simulink model "LQR_Luenberger_Hardware"  (R2021a)
settings: Solver=FixedStepAuto  StartTime=0.0  StopTime=100  FixedStep=0.002  RelTol=1e-3  EnableMultiTasking=on
undefined symbols (not defined in the file): K_lqr
libraries: simulink_extras x2, cstblocks x1
settings Model: ExtModeTrigDuration=10000  Creator=ACSI-MLC  LastModifiedBy=jameshong
settings SolverCC: AlgebraicLoopSolver=TrustRegion  PositivePriorityOrder=on
settings DataIOCC: ReturnWorkspaceOutputs=off
settings DebuggingCC: SFMachineParentedDataDiag=warning  ArithmeticOperatorsInVariantConditions=warning
settings SFSimCC: CustomCodeUndefinedFunction=UseInterfaceOnly
settings RTWCC: Description=QUARC Win64 Target  SystemTargetFile=quarc_win64.tlc  TemplateMakefile=quarc_default_tmf
settings STFCustomTargetCC: TargetPreCompLibLocation=C:\PROGRA~3\QUARC\lib\2018b\win64\release  TargetLangStandard=C99 (ISO)  ConcurrentExecutionCompliant=on  UseToolchainInfoCompliant=off  SystemTargetFile=quarc_win64.tlc
settings GRTTargetCC: TargetPreCompLibLocation=C:\PROGRA~3\QUARC\lib\2018b\win64\release  ParMdlRefBuildCompliant=off  CompOptLevelCompliant=off  CombineOutputUpdateFcns=off  MatFileLogging=off  CPPClassGenCompliant=off  GRTInterface=on  UseToolchainInfoCompliant=off  ExtMode=on  ExtModeMexFile=quarc_comm

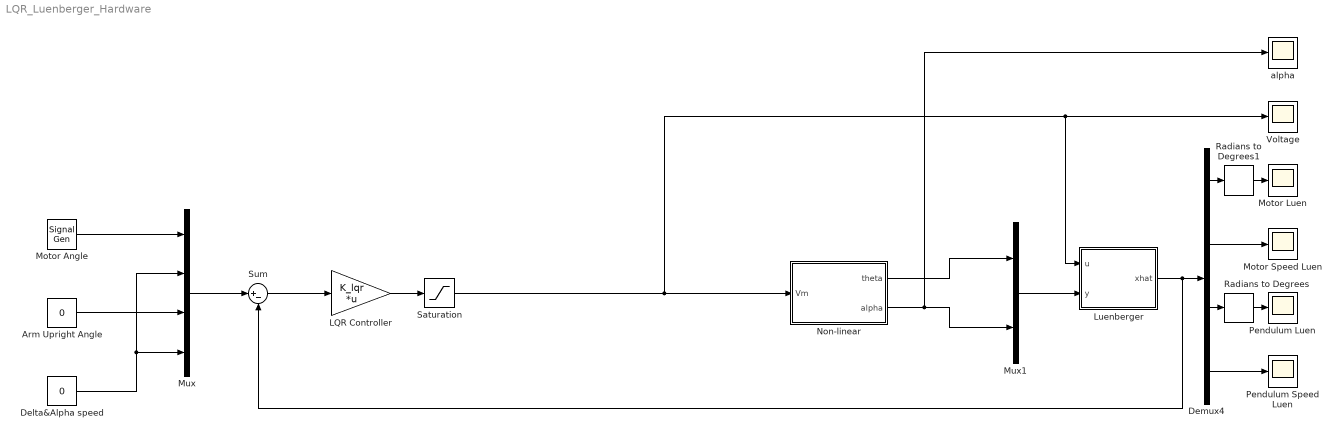
== system LQR_Luenberger_Hardware ==
  Arm Upright Angle : Constant  Value=0
  Delta&Alpha speed : Constant  Value=0
  Demux4 : Demux
  LQR Controller : Gain  Gain=K_lqr  Multiplication=Matrix(K*u) (u vector)
  Luenberger : Subsystem
  Motor Angle : SignalGenerator  WaveForm=square  Amplitude=30/180*pi  Frequency=0.2
  Motor Luen : Scope
  Motor Speed Luen : Scope
  Mux : Mux
  Mux1 : Mux  Inputs=2
  Non-linear : Subsystem
  Pendulum Luen : Scope
  Pendulum Speed Luen : Scope
  Radians to Degrees : simulink_extras/Transformations/Radians to Degrees
  Radians to Degrees1 : simulink_extras/Transformations/Radians to Degrees
  Saturation : Saturate  UpperLimit=24  LowerLimit=-24
  Sum : Sum  Inputs=|+-
  Voltage : Scope
  alpha : Scope
  wires:
  Demux4/1 -> Radians to Degrees1/1
  Luenberger/1(xhat) -> Sum/2, Demux4/1
  Mux1/1 -> Luenberger/2(y)
  Sum/1 -> LQR Controller/1
  LQR Controller/1 -> Saturation/1
  Delta&Alpha speed/1 -> Mux/4, Mux/2
  Demux4/4 -> Pendulum Speed Luen/1
  Arm Upright Angle/1 -> Mux/3
  Demux4/3 -> Radians to Degrees/1
  Demux4/2 -> Motor Speed Luen/1
  Mux/1 -> Sum/1
  Saturation/1 -> Non-linear/1(Vm), Luenberger/1(u), Voltage/1
  Non-linear/1(theta) -> Mux1/1
  Non-linear/2(alpha) -> alpha/1, Mux1/2
  Radians to Degrees/1 -> Pendulum Luen/1
  Radians to Degrees1/1 -> Motor Luen/1
  Motor Angle/1 -> Mux/1

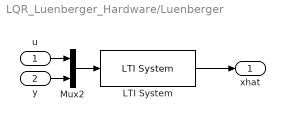
== system LQR_Luenberger_Hardware/Luenberger ==
  u : Inport
  y : Inport  Port=2
  LTI System : cstblocks/LTI System  sys=obs_luen  IC=[0, 0, 0, 0]
  Mux2 : Mux  Inputs=2
  xhat : Outport
  wires:
  Mux2/1 -> LTI System/1
  LTI System/1 -> xhat/1
  y/1 -> Mux2/2
  u/1 -> Mux2/1

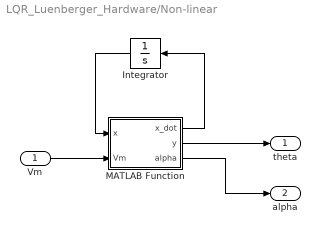
== system LQR_Luenberger_Hardware/Non-linear ==
  Vm : Inport
  Integrator : Integrator  InitialCondition=[0 0 pi/6 0]
  MATLAB Function : MATLAB Function  TreatAsAtomicUnit=on
  theta : Outport
  alpha : Outport  Port=2
  wires:
  MATLAB Function/1(x_dot) -> Integrator/1
  MATLAB Function/2(y) -> theta/1
  Integrator/1 -> MATLAB Function/1(x)
  Vm/1 -> MATLAB Function/2(Vm)
  MATLAB Function/3(alpha) -> alpha/1

== matlab function LQR_Luenberger_Hardware/Non-linear/MATLAB Function ==
  data: x input; x_dot output; Vm input; y output; alpha output
function [x_dot, y, alpha] = fcn(x, Vm)
x_dot = [x(2); get_theta_ddot(x(1),x(2),x(3),x(4),Vm); x(4); get_alpha_ddot(x(1),x(2),x(3),x(4),Vm)];
y = x(1);
alpha = x(3);
end
